simulink model "lift"  (R2024b)
settings: Solver=VariableStepAuto  StartTime=0.0  StopTime=inf  RelTol=1e-3
settings Model: Creator=Ajay1  LastModifiedBy=Ajay1

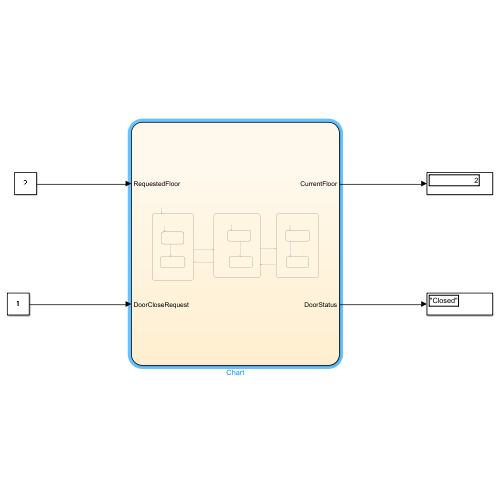
[thumbnail: Simulink's stored preview of the top-level diagram]
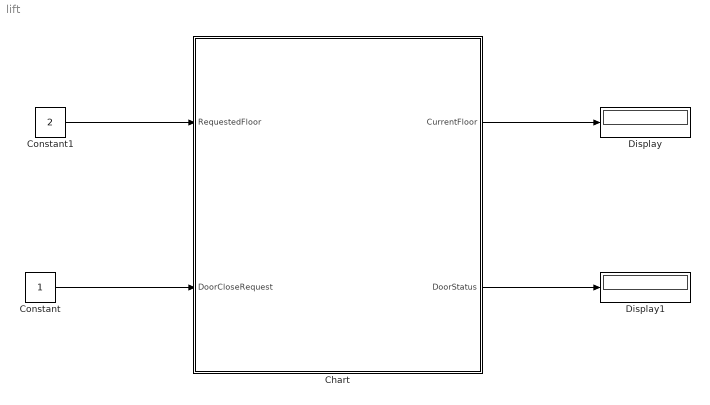
== system lift ==
  Chart : Stateflow chart  TreatAsAtomicUnit=on
  Constant : Constant
  Constant1 : Constant  Value=2
  Display : Display
      settings: Decimation=2
  Display1 : Display
  wires:
  Constant/1 -> Chart/2(DoorCloseRequest)
  Chart/1(CurrentFloor) -> Display/1
  Chart/2(DoorStatus) -> Display1/1
  Constant1/1 -> Chart/1(RequestedFloor)

== stateflow chart lift/Chart ==
  state floor1
    entry:
    CurrentFloor = 1;
    state dooropened
      entry:
      DoorStatus = "Open";
    state doorclosed
      entry:
      DoorStatus = "Closed";
    (default) -> floor1.dooropened
    floor1.dooropened -> floor1.doorclosed : [DoorCloseRequest]
  state floor2
    entry:
    CurrentFloor = 2;
    state dooropened
      entry:
      DoorStatus = "Open";
    state doorclosed
      entry:
      DoorStatus = "Closed";
    (default) -> floor2.dooropened
    floor2.dooropened -> floor2.doorclosed : [DoorCloseRequest]
  state floor3
    entry:
    CurrentFloor = 3;
    state dooropened
      entry:
      DoorStatus = "Open";
    state doorclosed
      entry:
      DoorStatus = "Closed";
    (default) -> floor3.dooropened
    floor3.dooropened -> floor3.doorclosed : [DoorCloseRequest]
  (default) -> floor1
  floor2 -> floor3 [order 1] : [RequestedFloor == 3 &&...
      |  DoorStatus == "Closed"]
  floor1 -> floor2 : [RequestedFloor ~= 1 &&...
      |  DoorStatus == "Closed"]
  floor2 -> floor1 [order 2] : [RequestedFloor == 1 &&...
      |  DoorStatus == "Closed"]
  floor3 -> floor2 : [RequestedFloor == 2 &&...
      |  DoorStatus == "Closed"]
  data: RequestedFloor input; DoorCloseRequest input; CurrentFloor output; DoorStatus output string
